simulink model "sfcndemo_sfun_multirate"  (Simulink 7.6)
settings: Solver=FixedStepDiscrete  StartTime=0.0  StopTime=5  RelTol=1e-3
Description:
  | Multirate C-MEX S-function
settings Model: Creator=The MathWorks Inc.  ExtModeTrigMode=oneshot  ExtModeArmWhenConnect=off  ExtModeAutoUpdateStatusClock=off
settings DataIOCC: LimitDataPoints=off  SaveState=on
settings OptimizationCC: BooleanDataType=off  InlineInvariantSignals=on  InitFltsAndDblsToZero=on
settings DebuggingCC: SaveWithParameterizedLinksMsg=none  SignalResolutionControl=TryResolveAllWithWarning  SolverPrmCheckMsg=none  InheritedTsInSrcMsg=none  MultiTaskDSMMsg=warning  MultiTaskCondExecSysMsg=none  UnconnectedInputMsg=none  UnconnectedOutputMsg=none
settings HardwareCC: TargetUnknown=on
settings RTWCC: IncludeERTFirstTime=on
settings CodeAppCC: CustomSymbolStrFcn=$F$N$M
settings GRTTargetCC: TargetFcnLib=ansi_tfl_tmw.mat

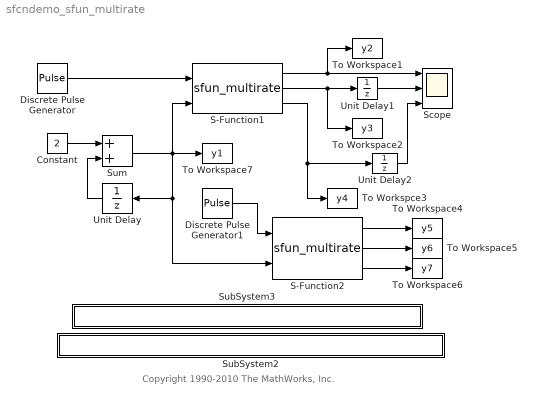
== system sfcndemo_sfun_multirate ==
  note: Copyright 1990-2010 The MathWorks, Inc.
  Constant : Constant  Value=2
  Discrete Pulse Generator : DiscretePulseGenerator  Period=100  PulseWidth=50  SampleTime=.01
  Discrete Pulse Generator1 : DiscretePulseGenerator  Period=100  PulseWidth=50  SampleTime=.1
  S-Function1 : S-Function  FunctionName=sfun_multirate  Parameters=k1,k2,k3  EnableBusSupport=off  mask(S-function: sfun_multirate){k1=2, k2=4, k3=8}
      mask prompts: k1 "First output rate"; k2 "Second output rate"; k3 "Third output rate"
      mask help: This is a multiple port, multi-rate S-function example. It accepts two input signals and produces three outputs.
  S-Function2 : S-Function  FunctionName=sfun_multirate  Parameters=k1,k2,k3  EnableBusSupport=off  mask(S-function: sfun_multirate){k1=2, k2=4, k3=8}
      mask prompts: k1 "First output rate"; k2 "Second output rate"; k3 "Third output rate"
      mask help: This is a multiple port, multi-rate S-function example. It accepts two input signals and produces three outputs.
  Scope : Scope  NumInputPorts=3
      settings: TimeRange=5  YMin=0~0~0  YMax=120~100~100
  SubSystem2 : Subsystem  mask{filename=sfun_multirate.tlc}
      mask init:
      | x=sfundemo_maskdisp;
      settings: AttributesFormatString=\n  OpenFcn=sfundemo_openfcn
      mask Display: disp(x);
  SubSystem3 : Subsystem  mask{filename=sfun_multirate.c}
      mask init:
      | x=sfundemo_maskdisp;
      settings: AttributesFormatString=\n  OpenFcn=sfundemo_openfcn
      mask Display: disp(x);
  Sum : Sum  SaturateOnIntegerOverflow=on  InputSameDT=on  OutDataTypeStr=Inherit: Same as first input
  To Workspace1 : ToWorkspace  VariableName=y2  SampleTime=-1  SaveFormat=Structure With Time
  To Workspace2 : ToWorkspace  VariableName=y3  SampleTime=-1  SaveFormat=Structure With Time
  To Workspace4 : ToWorkspace  VariableName=y5  SampleTime=-1  SaveFormat=Structure With Time
  To Workspace5 : ToWorkspace  VariableName=y6  SampleTime=-1  SaveFormat=Structure With Time
  To Workspace6 : ToWorkspace  VariableName=y7  SampleTime=-1  SaveFormat=Structure With Time
  To Workspace7 : ToWorkspace  VariableName=y1  SampleTime=-1  SaveFormat=Structure With Time
  To Workspce3 : ToWorkspace  VariableName=y4  SampleTime=-1  SaveFormat=Structure With Time
  Unit Delay : UnitDelay  SampleTime=.1
  Unit Delay1 : UnitDelay  SampleTime=-1
  Unit Delay2 : UnitDelay  SampleTime=-1
  wires:
  Discrete Pulse Generator/1 -> S-Function1/1
  Sum/1 -> S-Function1/2, Unit Delay/1, S-Function2/2, To Workspace7/1
  Constant/1 -> Sum/1
  Unit Delay/1 -> Sum/2
  Discrete Pulse Generator1/1 -> S-Function2/1
  S-Function2/1 -> To Workspace4/1
  S-Function2/2 -> To Workspace5/1
  S-Function2/3 -> To Workspace6/1
  S-Function1/1 -> Scope/1, To Workspace1/1
  S-Function1/2 -> Unit Delay1/1, To Workspace2/1
  Unit Delay1/1 -> Scope/2
  Unit Delay2/1 -> Scope/3
  S-Function1/3 -> Unit Delay2/1, To Workspce3/1

== system sfcndemo_sfun_multirate/SubSystem2 ==

== system sfcndemo_sfun_multirate/SubSystem3 ==
